simulink library "aircraft_refuel_control"  (R2024b)
settings: Solver=VariableStepAuto  StartTime=0.0  StopTime=10.0  RelTol=1e-3
undefined symbols (not defined in the file): ABORT_MODE, CHILLDOWN, CLOSE, CONNECTED, DEFUEL, DEFUEL_MODE, DISCONNECTED, FEED, IDLE, OPEN, REFUEL, REFUEL_MODE, timestep, WARMUP
settings Model: Creator=MW  LastModifiedBy=MW

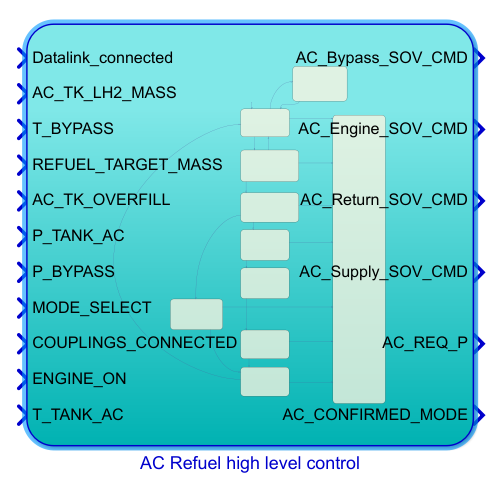
[thumbnail: Simulink's stored preview of the top-level diagram]
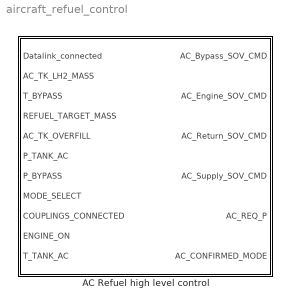
== system aircraft_refuel_control ==
  AC Refuel high level control : Stateflow chart  TreatAsAtomicUnit=on  SystemSampleTime=timestep

== stateflow chart aircraft_refuel_control/AC Refuel high level control ==
  state ENGINE_FEED
    en, du:
    AC_REQ_P = 0.11;
    AC_Bypass_SOV_CMD = CLOSE;
    AC_Supply_SOV_CMD = CLOSE;
    AC_Return_SOV_CMD = CLOSE;
    AC_Engine_SOV_CMD = OPEN;
    AC_CONFIRMED_MODE = FEED;
  state IDLE
    en, du:
    AC_REQ_P = 0.11;
    AC_Bypass_SOV_CMD = CLOSE;
    AC_Supply_SOV_CMD = CLOSE;
    AC_Return_SOV_CMD = CLOSE;
    AC_Engine_SOV_CMD = CLOSE;
    AC_CONFIRMED_MODE = IDLE;
  state EMERGENCY_STOP
    en:
    AC_Bypass_SOV_CMD = OPEN;
    AC_Supply_SOV_CMD = CLOSE;
    AC_Return_SOV_CMD = CLOSE;
    AC_Engine_SOV_CMD = CLOSE;
    AC_CONFIRMED_MODE = ABORT_MODE;
  state CHECK_INTEGRITY
    en, du:
    AC_REQ_P = 0.11;
    AC_Bypass_SOV_CMD = CLOSE;
    AC_Supply_SOV_CMD = CLOSE;
    AC_Return_SOV_CMD = CLOSE;
    AC_Engine_SOV_CMD = CLOSE;
    confirmed_mode = MODE_SELECT;
  state CHILLDOWN
    en, du:
    AC_REQ_P = P_BYPASS;
    AC_Bypass_SOV_CMD = OPEN;
    AC_Supply_SOV_CMD = CLOSE;
    AC_Return_SOV_CMD = CLOSE;
    AC_Engine_SOV_CMD = CLOSE;
    AC_CONFIRMED_MODE = CHILLDOWN;
  state TANK_FILL
    en, du:
    AC_REQ_P = P_TANK_AC;
    AC_Bypass_SOV_CMD = CLOSE;
    AC_Supply_SOV_CMD = OPEN;
    AC_Return_SOV_CMD = OPEN;
    AC_Engine_SOV_CMD = CLOSE;
    AC_CONFIRMED_MODE = REFUEL;
  state TANK_SOAK
    en, du:
    AC_REQ_P = P_TANK_AC;
    AC_Bypass_SOV_CMD = CLOSE;
    AC_Supply_SOV_CMD = CLOSE;
    AC_Return_SOV_CMD = OPEN;
    AC_Engine_SOV_CMD = CLOSE;
    AC_CONFIRMED_MODE = REFUEL;
  state TANK_DRAIN
    en, du:
    AC_REQ_P = P_TANK_AC;
    AC_Bypass_SOV_CMD = CLOSE;
    AC_Supply_SOV_CMD = OPEN;
    AC_Return_SOV_CMD = OPEN;
    AC_Engine_SOV_CMD = CLOSE;
    AC_CONFIRMED_MODE = DEFUEL;
  state WARMUP
    en, du:
    AC_REQ_P = P_BYPASS;
    AC_Bypass_SOV_CMD = OPEN;
    AC_Supply_SOV_CMD = CLOSE;
    AC_Return_SOV_CMD = CLOSE;
    AC_Engine_SOV_CMD = CLOSE;
    AC_CONFIRMED_MODE = WARMUP;
  state DISCONNECT
    en, du:
    AC_REQ_P = 0.11;
    AC_Bypass_SOV_CMD = CLOSE;
    AC_Supply_SOV_CMD = CLOSE;
    AC_Return_SOV_CMD = CLOSE;
    AC_Engine_SOV_CMD = CLOSE;
    AC_CONFIRMED_MODE = DISCONNECT;
  IDLE -> ENGINE_FEED [order 3] : [ENGINE_ON && ...
      | Datalink_connected  == DISCONNECTED && ...
      | COUPLINGS_CONNECTED == DISCONNECTED]
  ENGINE_FEED -> IDLE : [~ENGINE_ON || ...
      | ~(Datalink_connected  == DISCONNECTED && ...
      | COUPLINGS_CONNECTED == DISCONNECTED)]
  (default) -> IDLE
  IDLE -> EMERGENCY_STOP [order 1] : [AC_TK_OVERFILL]
  DISCONNECT -> IDLE [order 2] : [Datalink_connected  == DISCONNECTED && ...
      | COUPLINGS_CONNECTED == DISCONNECTED]
  IDLE -> CHECK_INTEGRITY [order 2] : [Datalink_connected == CONNECTED]
  CHECK_INTEGRITY -> IDLE [order 3] : [Datalink_connected  == DISCONNECTED]
  CHECK_INTEGRITY -> EMERGENCY_STOP [order 1] : [AC_TK_OVERFILL]
  CHECK_INTEGRITY -> CHILLDOWN [order 2] : [Datalink_connected == CONNECTED && ...
      | COUPLINGS_CONNECTED == CONNECTED]
  CHILLDOWN -> EMERGENCY_STOP [order 1] : [AC_TK_OVERFILL]
  CHILLDOWN -> TANK_DRAIN [order 3] : [T_BYPASS < 30 && ...
      | confirmed_mode == DEFUEL_MODE]
  CHILLDOWN -> TANK_FILL [order 2] : [T_BYPASS < 30 && ...
      | confirmed_mode == REFUEL_MODE]
  TANK_SOAK -> TANK_FILL [order 2] : after(10, sec)
      | [REFUEL_TARGET_MASS - AC_TK_LH2_MASS ...
      | >= GAUGE_ERROR]
  TANK_FILL -> EMERGENCY_STOP [order 1] : [AC_TK_OVERFILL]
  TANK_FILL -> TANK_SOAK [order 2] : [AC_TK_LH2_MASS >= REFUEL_TARGET_MASS]
  TANK_SOAK -> WARMUP [order 1] : after(10, sec)
      | [REFUEL_TARGET_MASS - AC_TK_LH2_MASS ...
      | <= GAUGE_ERROR]
  TANK_DRAIN -> EMERGENCY_STOP [order 1] : [AC_TK_OVERFILL]
  TANK_DRAIN -> DISCONNECT [order 2] : [REFUEL_TARGET_MASS <= 1 && ...
      | T_BYPASS > 270]
  WARMUP -> EMERGENCY_STOP [order 1] : [AC_TK_OVERFILL]
  WARMUP -> DISCONNECT [order 2] : [T_BYPASS > 270]
  DISCONNECT -> EMERGENCY_STOP [order 1] : [AC_TK_OVERFILL]
  data: Datalink_connected input; AC_TK_LH2_MASS input; T_BYPASS input; REFUEL_TARGET_MASS input; AC_Bypass_SOV_CMD output; AC_Engine_SOV_CMD output; AC_Return_SOV_CMD output; AC_Supply_SOV_CMD output; CLOSE parameter; OPEN parameter; AC_TK_OVERFILL input; P_TANK_AC input; AC_REQ_P output; P_BYPASS input; MODE_SELECT input; REFUEL parameter; DEFUEL parameter; AC_CONFIRMED_MODE output; confirmed_mode local; IDLE parameter; CHILLDOWN parameter; WARMUP parameter; DEFUEL_MODE parameter; REFUEL_MODE parameter; COUPLINGS_CONNECTED input; CONNECTED parameter; DISCONNECTED parameter; FEED parameter; ENGINE_ON input; ABORT_MODE parameter; T_TANK_AC input; GAUGE_ERROR constant double =0.1
